simulink model "sm_robot_6legs_4bar"  (R2026a)
settings: Solver=ode15s  StopTime=33  MaxStep=1e-1  AbsTol=1e-4  EnableMultiTasking=on
PostLoadFcn:
  | sm_robot_6legs_4bar_param
undefined symbols (not defined in the file or in its folder): flr1_dep, flr1_len, flr1_wid, flr2_ang, flr2_dep, flr2_len, flr2_wid, flr3_dep, flr3_len, flr3_wid, flr_dep_pcnt, link_h, sigbuilder_block, X, Y, Z
libraries: Contact_Forces_Lib x24, sm_lib x12, nesl_utility x5, sm_robot_6legs_4bar_lib x2
CloseFcn:
  | try,close(h1_sm_robot_6legs_4bar),end
  | clear h1_sm_robot_6legs_4bar
  | 
  | clear simlog_sm_robot_6legs_4bar
  | clear logsout_sm_robot_6legs_4bar
Description:
  | Robot with Six Legs Built From 4 Four-Bar Linkages
  | 
  | Copyright 2026 The MathWorks, Inc.
settings Model: Creator=smiller  LastModifiedBy=smiller
settings DataIOCC: MaxDataPoints=20000  SignalLoggingName=logsout_sm_robot_6legs_4bar
settings DebuggingCC: PregeneratedLibrarySubsystemCodeDiagnostic=none
settings SimscapeCC: SimscapeNominalValues="[{\"value\":\"10\",\"unit\":\"V\"},{\"value\":\"1\",\"unit\":\"A\"},{\"value\":\"10\",\"unit\":\"N*m\"},{\"value\":\"10\",\"unit\":\"bar\"},{\"value\":\"100\",\"unit\":\"kJ/kg\"},{\"value\":\"1\",\"unit\":\"kW\"},{\"value\":\"300\",\"unit\":\"K\"},{\"value\":\"100\",\"unit\":\"cm^3/s\"},{\"value\":\"1\",\"unit\":\"kN\"},{\"value\":\"1\",\"unit\":\"g/cm^3\"},{\"value\":\"1\",\"unit\":\"l\"},{\"value\":\"1\",\"unit\":\"cm^2\"},{\"value\":\"60\",\"unit\":\"Hz\"}]"  SimscapeLogSimulationStatistics=on  SimscapeLogName=simlog_sm_robot_6legs_4bar  SimscapeLogDataHistory=20000.0
settings ConfigurationSet: Description=SimMechanics 2G
settings DiagnosticsConfigSet: SimMechanicsRigidlyBoundBlock=none
settings ExplorerConfigSet: InternalSimMechanicsExplorerSettings="<ExplorerConfiguration><canonicalview>default</canonicalview><AnimationSetting><BasePlaybackSpeed>1.0</BasePlaybackSpeed><PlaybackSpeedFactor>1.0</PlaybackSpeedFactor></AnimationSetting><TilePanel><TileInfo><Tiles Columns=\"2\" Count=\"3\" Rows=\"2\"><Column Weight=\"0.7315\"/><Column Weight=\"0.2685\"/><Row Weight=\"0.3085\"/><Row Weight=\"0.6915\"/><Tile Height=\"1\" Width=\"2\" X=\"0\" Y=\"0\"/><Tile Height=\"1\" Width=\"1\" X=\"0\" Y=\"1\"/><Tile Height=\"1\" Width=\"1\" X=\"1\" Y=\"1\"/></Tiles></TileInfo><SceneInfo><SceneViewer><BGColor><R>1</R><G>1</G><B>1</B></BGColor><Camera><DoPerspective>off</DoPerspective><Position><X>0.0595264996404310034</X><Y>0.0499787248889781988</Y><Z>-1.00000003287775163</Z></Position><Center><X>0.0595264996404310034</X><Y>0.0499787248889781988</Y><Z>-3.28777516322986685e-08</Z></Center><Up><X>0.00262045319823715674</X><Y>0.999996566606623727</Y><Z>0</Z></Up><ViewLimDist>1</ViewLimDist><YLim>0.107978090662275067</YLim><XLim>0.373654416059221617</XLim></Camera></SceneViewer><SceneViewer><BGColor><R>1</R><G>1</G><B>1</B></BGColor><Camera><DoPerspective>off</DoPerspective><Position><X>-0.747368609679726625</X><Y>0.501177725000622964</Y><Z>-0.454021615890128183</Z></Position><Center><X>0.0441835460138454428</X><Y>0.0596697074532213934</Y><Z>-0.0315102488735390512</Z></Center><Up><X>0.430303060009063654</X><Y>0.893614327868432756</Y><Z>0.127642898647299968</Z></Up><ViewLimDist>1</ViewLimDist><YLim>0.188959781718016667</YLim><XLim>0.209955313020018519</XLim></Camera></SceneViewer><SceneViewer><BGColor><R>1</R><G>1</G><B>1</B></BGColor><Camera><DoPerspective>off</DoPerspective><Position><X>0.0495837117205682534</X><Y>1.05623067821298733</Y><Z>0.0484295084377242974</Z></Position><Center><X>0.0433038677712018413</X><Y>0.0567676171677271926</Y><Z>0.0162712565261088245</Z></Center><Up><X>0.999975191574708711</X><Y>-0.00637917136590451708</Y><Z>0.00298703997456827193</Z></Up><ViewLimDist>1</ViewLimDist><YLim>0.384512045360850374</YLim><XLim>0.15427952437318071</XLim></Camera></SceneViewer></SceneInfo></TilePanel><MechEditorPanel><Cameras/><GfxPanelCameraMap/><VideoCreator><PlaybackSpeedRatio>2.0</PlaybackSpeedRatio><FrameRate>30</FrameRate><VideoFormat>MPEG-4</VideoFormat><FrameSize>auto</FrameSize></VideoCreator></MechEditorPanel></ExplorerConfiguration>"

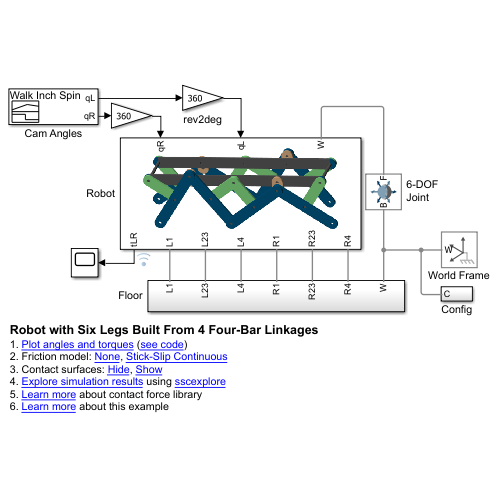
[thumbnail: Simulink's stored preview of the top-level diagram]
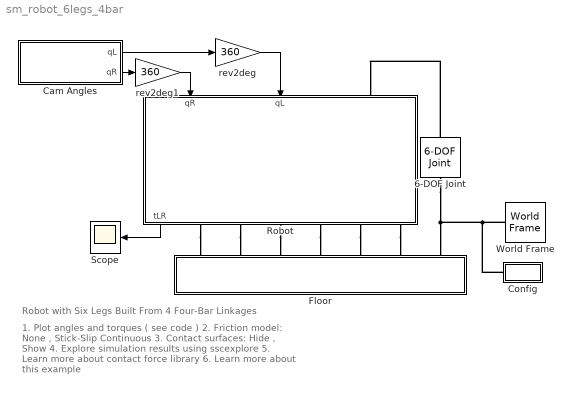
== system sm_robot_6legs_4bar ==
  note: Robot with Six Legs Built From 4 Four-Bar Linkages
  note: 1. Plot angles and torques ( see code )
      | 2. Friction model: None , Stick-Slip Continuous
      | 3. Contact surfaces: Hide , Show
      | 4. Explore simulation results using sscexplore
      | 5. Learn more about contact force library
      | 6. Learn more about this example
  6-DOF Joint : sm_lib/Joints/6-DOF Joint  JointMode=Normal  CompositeWrenchDir=FollowerOnBase  CompositeWrenchFrame=BaseFrame  SenseConstraintForce=off  SenseConstraintTorque=off  SenseTotalForce=off  SenseTotalTorque=off  PxPositionTargetSpecify=on  PxPositionTargetPriority=High  PxPositionTargetValue=-flr1_len/4-4.1e-2  PxPositionTargetValueUnits=m  PxVelocityTargetSpecify=off  PxVelocityTargetPriority=High  PxVelocityTargetValue=0  PxVelocityTargetValueUnits=m/s  PxEquilibriumPosition=0  PxEquilibriumPositionUnits=m  PxSpringStiffness=0  PxSpringStiffnessUnits=N/m  PxDampingCoefficient=0  PxDampingCoefficientUnits=N/(m/s)  PxLowerLimitSpecify=off  PxLowerLimitBound=-1  PxLowerLimitBoundUnits=m  PxLowerLimitStiffness=1e6  PxLowerLimitStiffnessUnits=N/m  PxLowerLimitDamping=1e3  PxLowerLimitDampingUnits=N/(m/s)  PxLowerLimitTransitionRegionWidth=1e-4  PxLowerLimitTransitionRegionWidthUnits=m  PxUpperLimitSpecify=off  PxUpperLimitBound=1  PxUpperLimitBoundUnits=m  PxUpperLimitStiffness=1e6  PxUpperLimitStiffnessUnits=N/m  PxUpperLimitDamping=1e3  PxUpperLimitDampingUnits=N/(m/s)  PxUpperLimitTransitionRegionWidth=1e-4  PxUpperLimitTransitionRegionWidthUnits=m  PxTorqueActuationMode=NoTorque  PxMotionActuationMode=ComputedMotion  PxSensePosition=off  PxSenseVelocity=off  PxSenseAcceleration=off  PxSenseTorqueForce=off  PxSenseLowerLimitTorqueForce=off  PxSenseUpperLimitTorqueForce=off  PyPositionTargetSpecify=on  PyPositionTargetPriority=High  PyPositionTargetValue=leg_l  PyPositionTargetValueUnits=m  PyVelocityTargetSpecify=off  PyVelocityTargetPriority=High  PyVelocityTargetValue=0  PyVelocityTargetValueUnits=m/s  PyEquilibriumPosition=0  PyEquilibriumPositionUnits=m  PySpringStiffness=0  PySpringStiffnessUnits=N/m  PyDampingCoefficient=0  PyDampingCoefficientUnits=N/(m/s)  PyLowerLimitSpecify=off  PyLowerLimitBound=-1  PyLowerLimitBoundUnits=m  PyLowerLimitStiffness=1e6  PyLowerLimitStiffnessUnits=N/m  PyLowerLimitDamping=1e3  PyLowerLimitDampingUnits=N/(m/s)  PyLowerLimitTransitionRegionWidth=1e-4  PyLowerLimitTransitionRegionWidthUnits=m  PyUpperLimitSpecify=off  PyUpperLimitBound=1  PyUpperLimitBoundUnits=m  PyUpperLimitStiffness=1e6  PyUpperLimitStiffnessUnits=N/m  PyUpperLimitDamping=1e3  PyUpperLimitDampingUnits=N/(m/s)  PyUpperLimitTransitionRegionWidth=1e-4  PyUpperLimitTransitionRegionWidthUnits=m  PyTorqueActuationMode=NoTorque  PyMotionActuationMode=ComputedMotion  PySensePosition=off  PySenseVelocity=off  PySenseAcceleration=off  PySenseTorqueForce=off  PySenseLowerLimitTorqueForce=off  PySenseUpperLimitTorqueForce=off  PzPositionTargetSpecify=off  PzPositionTargetPriority=High  PzPositionTargetValue=0  PzPositionTargetValueUnits=m  PzVelocityTargetSpecify=off  PzVelocityTargetPriority=High  PzVelocityTargetValue=0  PzVelocityTargetValueUnits=m/s  PzEquilibriumPosition=0  PzEquilibriumPositionUnits=m  PzSpringStiffness=0  PzSpringStiffnessUnits=N/m  PzDampingCoefficient=0  PzDampingCoefficientUnits=N/(m/s)  PzLowerLimitSpecify=off  PzLowerLimitBound=-1  PzLowerLimitBoundUnits=m  PzLowerLimitStiffness=1e6  PzLowerLimitStiffnessUnits=N/m  PzLowerLimitDamping=1e3  PzLowerLimitDampingUnits=N/(m/s)  PzLowerLimitTransitionRegionWidth=1e-4  PzLowerLimitTransitionRegionWidthUnits=m  PzUpperLimitSpecify=off  PzUpperLimitBound=1  PzUpperLimitBoundUnits=m  PzUpperLimitStiffness=1e6  PzUpperLimitStiffnessUnits=N/m  PzUpperLimitDamping=1e3  PzUpperLimitDampingUnits=N/(m/s)  PzUpperLimitTransitionRegionWidth=1e-4  PzUpperLimitTransitionRegionWidthUnits=m  PzTorqueActuationMode=NoTorque  PzMotionActuationMode=ComputedMotion  PzSensePosition=off  PzSenseVelocity=off  PzSenseAcceleration=off  PzSenseTorqueForce=off  PzSenseLowerLimitTorqueForce=off  PzSenseUpperLimitTorqueForce=off  SphPositionTargetSpecify=off  SphPositionTargetPriority=High  SphPositionTargetRotationMethod=None  SphPositionTargetFollAlignAxisA=+X  SphPositionTargetBaseAlignAxisA=+Y  SphPositionTargetFollAlignAxisB=+Y  SphPositionTargetBaseAlignAxisB=+Z  SphPositionTargetRotationStandardAxis=+Z  SphPositionTargetRotationAngle=0.0  SphPositionTargetRotationAngleUnits=deg  SphPositionTargetRotationArbitraryAxis=[0 0 1]  SphPositionTargetRotationSequenceAxes=FollowerAxes  SphPositionTargetRotationSequence=XYX  SphPositionTargetRotationSequenceAngles=[0 0 0]  SphPositionTargetRotationSequenceAnglesUnits=deg  SphPositionTargetRotationMatrix=[1 0 0; 0 1 0; 0 0 1]  SphPositionTargetQuaternion=[1 0 0 0]  SphVelocityTargetSpecify=off  SphVelocityTargetPriority=High  SphVelocityTargetValue=[0 0 0]  SphVelocityTargetValueUnits=deg/s  SphVelocityTargetInFollowerFrame=on  SphEqPosRotationMethod=None  SphEqPosFollAlignAxisA=+X  SphEqPosBaseAlignAxisA=+Y  SphEqPosFollAlignAxisB=+Y  SphEqPosBaseAlignAxisB=+Z  SphEqPosRotationStandardAxis=+Z  SphEqPosRotationAngle=0.0  SphEqPosRotationAngleUnits=deg  SphEqPosRotationArbitraryAxis=[0 0 1]  SphEqPosRotationSequenceAxes=FollowerAxes  SphEqPosRotationSequence=XYX  SphEqPosRotationSequenceAngles=[0 0 0]  SphEqPosRotationSequenceAnglesUnits=deg  SphEqPosRotationMatrix=[1 0 0; 0 1 0; 0 0 1]  SphEqPosQuaternion=[1 0 0 0]  SphSpringStiffness=0  SphSpringStiffnessUnits=N*m/deg  SphDampingCoefficient=0  SphDampingCoefficientUnits=N*m/(deg/s)  SphLowerLimitSpecify=off  SphLowerLimitBound=15  SphLowerLimitBoundUnits=deg  SphLowerLimitStiffness=1e4  SphLowerLimitStiffnessUnits=N*m/deg  SphLowerLimitDamping=10  SphLowerLimitDampingUnits=N*m/(deg/s)  SphLowerLimitTransitionRegionWidth=0.1  SphLowerLimitTransitionRegionWidthUnits=deg  SphUpperLimitSpecify=off  SphUpperLimitBound=45  SphUpperLimitBoundUnits=deg  SphUpperLimitStiffness=1e4  SphUpperLimitStiffnessUnits=N*m/deg  SphUpperLimitDamping=10  SphUpperLimitDampingUnits=N*m/(deg/s)  SphUpperLimitTransitionRegionWidth=0.1  SphUpperLimitTransitionRegionWidthUnits=deg  SphTorqueActuationMode=NoTorque  SphActuateTorqueX=off  SphActuateTorqueY=off  SphActuateTorqueZ=off  SphActuateTorque=off  SphActuationFrame=BaseFrame  SphSensePosition=off  SphSenseVelocityX=off  SphSenseVelocityY=off  SphSenseVelocityZ=off  SphSenseVelocity=off  SphSenseAccelerationX=off  SphSenseAccelerationY=off  SphSenseAccelerationZ=off  SphSenseAcceleration=off  SphSenseLowerLimitTorqueMag=off  SphSenseUpperLimitTorqueMag=off  SphSensingFrame=BaseFrame
  Cam Angles : Subsystem  Tag=STV Subsys  LoadFcn=sigbuilder_block('load');  StartFcn=sigbuilder_block('start');  StopFcn=sigbuilder_block('stop');  ClipboardFcn=sigbuilder_block('clipboard');  mask(Sigbuilder block){tuvar=[0:10]}
      mask help: Simulink:masks:SigbuilderBlock_MD
      mask init:
      | if ~strcmp(get_param(bdroot(gcbh),'SimulationStatus'),'stopped') tuvar = sigbuilder_block('maskInit'); end
      settings: CopyFcn=sigbuilder_block('copy');  DeleteFcn=sigbuilder_block('delete');  ModelCloseFcn=sigbuilder_block('modelClose');  PreSaveFcn=sigbuilder_block('preSave');  PauseFcn=sigbuilder_block('pause');  ContinueFcn=sigbuilder_block('continue');  NameChangeFcn=sigbuilder_block('namechange');  OpenFcn=sigbuilder_block('open',[355.8 216 550.8 400.2 ]);  CloseFcn=sigbuilder_block('close');
      mask Display: plot(0, 0, 100, 100,[2, 2, 32, 32, 2], [68, 8, 8, 68, 68],[32, 2], [38, 38], [32, 19, 2],[53, 60, 44], [32, 17, 17, 2],[16, 16, 31, 31]);txt = getActiveGroup(gcbh);text(2, 100, txt,'verticalAlignment', 'top');
  Config : Subsystem
  Floor : Subsystem
  Robot : Subsystem  Tag=PublishSubsystem
      mask Display: image('sm_robot_6legs_4bar_robot_IMAGE.png')
  Scope : Scope
      settings: ActiveDisplayYMinimum=-0.58589  ActiveDisplayYMaximum=0.586
  World Frame : sm_lib/Frames and Transforms/World Frame
  rev2deg : Gain  Gain=360
  rev2deg1 : Gain  Gain=360
  wires:
  Cam Angles/2(qR) -> rev2deg1/1
  Cam Angles/1(qL) -> rev2deg/1
  Robot/1(tLR) -> Scope/1
  rev2deg/1 -> Robot/2(qL)
  rev2deg1/1 -> Robot/1(qR)
  connections:
  World Frame/RConn1 -- Config/LConn1 -- 6-DOF Joint/LConn1 -- Floor/LConn7
  6-DOF Joint/RConn1 -- Robot/LConn1
  Robot/RConn4 -- Floor/LConn4
  Robot/RConn5 -- Floor/LConn5
  Robot/RConn6 -- Floor/LConn6
  Robot/RConn1 -- Floor/LConn1
  Robot/RConn2 -- Floor/LConn2
  Robot/RConn3 -- Floor/LConn3

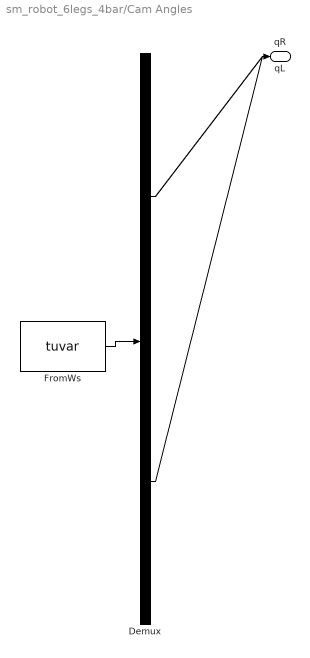
== system sm_robot_6legs_4bar/Cam Angles ==
  Demux : Demux  Tag=STV Demux  Outputs=2
      settings: DisplayOption=none
  FromWs : FromWorkspace  Tag=STV FromWs  VariableName=tuvar
      SigBuilderData=|
      | common.afterFinalStr = 'Extrapolate'
      | common.sampleTime = 0
      | dataSet(1).timeRange = [0 35]
      | dataSet(1).name = 'Walk Inch Spin'
      | dataSet(2).timeRange = [0 30]
      | dataSet(2).name = 'Walk'
      | dataSet(3).timeRange = [0 30]
      | dataSet(3).name = 'Inchworm'
      | sbobj.Groups(1).Name = 'Walk Inch Spin'
      | sbobj.Groups(1).Signals(1).Name = 'qL'
      | sbobj.Groups(1).Signals(1).XData = [0 0.5 3 3.5 5 5.5 25.5 26 28 28.5 32.5 35]
      | sbobj.Groups(1).Signals(1).YData = [0.75 0.75 1.75 1.75 2.25 2.25 12.25 12.25 12.75 12.75 14.75 14.75]
      | sbobj.Groups(1).Signals(2).Name = 'qR'
      | sbobj.Groups(1).Signals(2).XData = [0 0.5 3 5 5.5 25.5 28.5 32.5 35]
      | sbobj.Groups(1).Signals(2).YData = [0.25 0.25 1.25 1.25 1.25 11.25 11.25 9.25 9.25]
      | sbobj.Groups(1).TimeRange = [0 35]
      | sbobj.Groups(2).Name = 'Walk'
      | sbobj.Groups(2).Signals(1).Name = 'qL'
      | sbobj.Groups(2).Signals(1).XData = [0 1 22 30]
      | sbobj.Groups(2).Signals(1).YData = [0.75 0.75 11.75 11.75]
      | sbobj.Groups(2).Signals(2).Name = 'qR'
      | sbobj.Groups(2).Signals(2).XData = [0 1 22 30]
      | sbobj.Groups(2).Signals(2).YData = [0.25 0.25 11.25 11.25]
      | sbobj.Groups(2).TimeRange = [0 30]
      | sbobj.Groups(3).Name = 'Inchworm'
      | sbobj.Groups(3).Signals(1).Name = 'qL'
      | sbobj.Groups(3).Signals(1).XData = [0 1 22 30]
      | sbobj.Groups(3).Signals(1).YData = [0.75 0.75 11.75 11.75]
      | sbobj.Groups(3).Signals(2).Name = 'qR'
      | sbobj.Groups(3).Signals(2).XData = [0 1 22 30]
      | sbobj.Groups(3).Signals(2).YData = [0.75 0.75 11.75 11.75]
      | sbobj.Groups(3).TimeRange = [0 30]
  qL : Outport  Tag=STV Outport  VectorParamsAs1DForOutWhenUnconnected=off
  qR : Outport  Tag=STV Outport  Port=2  VectorParamsAs1DForOutWhenUnconnected=off
  wires:
  FromWs/1 -> Demux/1
  Demux/1 -> qL/1
  Demux/2 -> qR/1

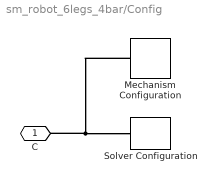
== system sm_robot_6legs_4bar/Config ==
  Mechanism Configuration : sm_lib/Utilities/Mechanism Configuration  UniformGravity=Constant  GravityVector=[0 -9.80665 0]  GravityVectorUnits=m/s^2  LinearizationDelta=0.001  JointModeTransitionNonlinearIterations=2
  Solver Configuration : nesl_utility/Solver Configuration  PhysicalDomain=network_engine_domain  SubClassName=solver  LeftPortType=input  RightPortType=generic  Tones=[]  Harmonics=[]  SimulateNoise=off  Profile=off  UseLocalSampling=off  EnableSwitchedLinearOptims=on  FrequencyDomain=off  UseCCode=off  RelTol=0.001  AbsTol=1e-06  MinStep=1e-09  ToWorkspace=off  RevertToSquareIcSolve=off  NumHomotopyIterations=100  PhasorMode=off  PhasorModeNumHarmonics=1  ConsistencySolver=NEWTON_FTOL  CanonicalOrdering=UNORDERED  OptimizeIntermediates=UNOPTIMIZED  IndexReductionMethod=DerivativeReplacement  DoDC=off  ResidualTolerance=1e-09  ConsistencyTolSource=GLOBAL  ConsistencyAbsTol=0.001  ConsistencyRelTol=0.001  ConsistencyTolFactor=0.001  UseLocalSolver=off  LocalSolverChoice=NE_BACKWARD_EULER_ADVANCER  ResolveIndetEquations=on  FunctionEvalNumThread=1  LocalSolverSampleTime=0.001  DoFixedCost=off  MaxNonlinIter=3  MaxModeIter=2  ComputeImpulses=off  ImpulseIterations=2  LinearAlgebra=Sparse  LinearAlgebraNumThread=0  EquationFormulation=NE_TIME_EF  DelaysMemoryBudget=1024  AutomaticFiltering=on  FilteringTimeConstant=0.001  PartitionStorageMethod=AS_NEEDED  PartitionMemoryBudget=1024  PartitionMethod=FAST  MultibodyUseLocalSolver=off  MultibodyLocalSolverChoice=ODE1  MultibodyLocalSolverSampleTime=0.001
  C : PMIOPort  Side=Left
  connections:
  Mechanism Configuration/RConn1 -- C/RConn1 -- Solver Configuration/RConn1

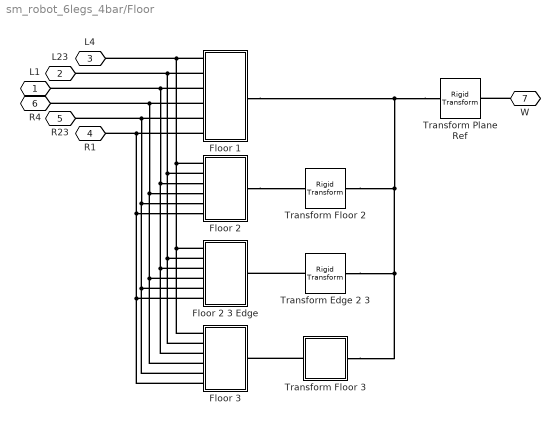
== system sm_robot_6legs_4bar/Floor ==
  Floor 1 : Subsystem  Tag=PublishSubsystem
  Floor 2 : Subsystem
  Floor 2 3 Edge : Subsystem
  Floor 3 : Subsystem
  Transform Edge 2 3 : sm_lib/Frames and Transforms/Rigid Transform  RotationMethod=AlignedAxes  FollAlignAxisA=+Z  BaseAlignAxisA=+Y  FollAlignAxisB=+X  BaseAlignAxisB=+Z  RotationStandardAxis=+Y  RotationAngle=-10  RotationAngleUnits=deg  RotationArbitraryAxis=[0 0 1]  RotationSequenceAxes=FollowerAxes  RotationSequence=XYX  RotationSequenceAngles=[0 0 0]  RotationSequenceAnglesUnits=deg  RotationMatrix=[1 0 0; 0 1 0; 0 0 1]  Quaternion=[1 0 0 0]  TranslationMethod=Cartesian  TranslationCartesianOffset=[cosd(flr2_ang) 0 sind(flr2_ang)]*flr2_len  TranslationCartesianOffsetUnits=m  TranslationStandardAxis=+Z  TranslationStandardOffset=0  TranslationStandardOffsetUnits=m  TranslationROffset=0  TranslationROffsetUnits=m  TranslationThetaOffset=0  TranslationThetaOffsetUnits=deg  TranslationZOffset=0  TranslationZOffsetUnits=m
  Transform Floor 2 : sm_lib/Frames and Transforms/Rigid Transform  RotationMethod=StandardAxis  FollAlignAxisA=+X  BaseAlignAxisA=+Y  FollAlignAxisB=+Y  BaseAlignAxisB=+Z  RotationStandardAxis=+Y  RotationAngle=-flr2_ang  RotationAngleUnits=deg  RotationArbitraryAxis=[0 0 1]  RotationSequenceAxes=FollowerAxes  RotationSequence=XYX  RotationSequenceAngles=[0 0 0]  RotationSequenceAnglesUnits=deg  RotationMatrix=[1 0 0; 0 1 0; 0 0 1]  Quaternion=[1 0 0 0]  TranslationMethod=Cartesian  TranslationCartesianOffset=[cosd(flr2_ang) 0 sind(flr2_ang)]*flr2_len/2  TranslationCartesianOffsetUnits=m  TranslationStandardAxis=+Z  TranslationStandardOffset=0  TranslationStandardOffsetUnits=m  TranslationROffset=0  TranslationROffsetUnits=m  TranslationThetaOffset=0  TranslationThetaOffsetUnits=deg  TranslationZOffset=0  TranslationZOffsetUnits=m
  Transform Floor 3 : Subsystem
  Transform Plane Ref : sm_lib/Frames and Transforms/Rigid Transform  RotationMethod=StandardAxis  FollAlignAxisA=+X  BaseAlignAxisA=+Y  FollAlignAxisB=+Y  BaseAlignAxisB=+Z  RotationStandardAxis=+X  RotationAngle=-90  RotationAngleUnits=deg  RotationArbitraryAxis=[0 0 1]  RotationSequenceAxes=FollowerAxes  RotationSequence=XYX  RotationSequenceAngles=[0 0 0]  RotationSequenceAnglesUnits=deg  RotationMatrix=[1 0 0; 0 1 0; 0 0 1]  Quaternion=[1 0 0 0]  TranslationMethod=None  TranslationCartesianOffset=[0 0 0]  TranslationCartesianOffsetUnits=m  TranslationStandardAxis=+Z  TranslationStandardOffset=0  TranslationStandardOffsetUnits=m  TranslationROffset=0  TranslationROffsetUnits=m  TranslationThetaOffset=0  TranslationThetaOffsetUnits=deg  TranslationZOffset=0  TranslationZOffsetUnits=m
  L1 : PMIOPort  Side=Left
  L23 : PMIOPort  Port=2  Side=Left
  L4 : PMIOPort  Port=3  Side=Left
  R1 : PMIOPort  Port=4  Side=Left
  R23 : PMIOPort  Port=5  Side=Left
  R4 : PMIOPort  Port=6  Side=Left
  W : PMIOPort  Port=7  Side=Left
  connections:
  W/RConn1 -- Transform Plane Ref/LConn1
  Floor 3/LConn1 -- Floor 2 3 Edge/LConn1 -- Floor 1/LConn1 -- L4/RConn1 -- Floor 2/LConn1
  Floor 3/LConn2 -- Floor 2 3 Edge/LConn2 -- Floor 1/LConn2 -- L23/RConn1 -- Floor 2/LConn2
  Floor 3/LConn3 -- Floor 2/LConn3 -- Floor 1/LConn3 -- L1/RConn1 -- Floor 2 3 Edge/LConn3
  R4/RConn1 -- Floor 1/LConn4 -- Floor 2 3 Edge/LConn4 -- Floor 3/LConn4 -- Floor 2/LConn4
  Transform Plane Ref/RConn1 -- Floor 1/RConn1 -- Transform Floor 3/LConn1 -- Transform Edge 2 3/LConn1 -- Transform Floor 2/LConn1
  R23/RConn1 -- Floor 1/LConn5 -- Floor 2 3 Edge/LConn5 -- Floor 3/LConn5 -- Floor 2/LConn5
  Floor 3/LConn6 -- Floor 2 3 Edge/LConn6 -- Floor 1/LConn6 -- R1/RConn1 -- Floor 2/LConn6
  Floor 2/RConn1 -- Transform Floor 2/RConn1
  Transform Floor 3/RConn1 -- Floor 3/RConn1
  Transform Edge 2 3/RConn1 -- Floor 2 3 Edge/RConn1

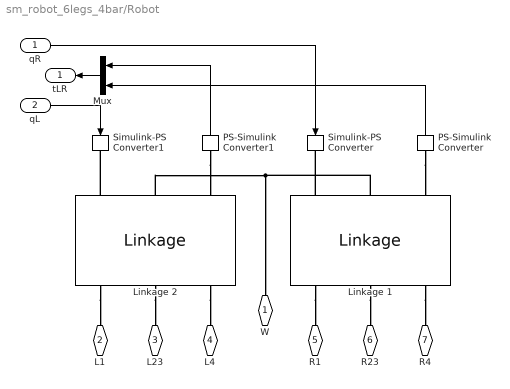
== system sm_robot_6legs_4bar/Robot ==
  qR : Inport
  qL : Inport  Port=2
  Linkage 1 : sm_robot_6legs_4bar_lib/Linkage  popup_LorR=Right
      link override Cam L12/Rod: popup_zori=Local +Z
      link override Cam L34/Rod: popup_zori=Local +Z
      link override Frame/Rod F1: popup_zori=Local +Z
      link override Frame/Rod F5: popup_zori=Local +Z
      link override Frame/Rod H1: popup_zori=Local +Z
      link override Frame/Rod H2: popup_zori=Local +Z
      link override Frame/Rod H4: popup_zori=Local +Z
      link override Frame/Rod H5: popup_zori=Local +Z
      link override Frame/Rod5 H3: popup_zori=Local +Z
      link override Leg L1/Rod: popup_zori=Local +Z
      link override Leg L3/Rod B: popup_zori=Local +Z
      link override Leg L3/Rod C: popup_zori=Local +Z
      link override Leg L3/Rod F: popup_zori=Local +Z
      link override Link L1/Rod: popup_zori=Local +Z
      link override Link L2/Rod: popup_zori=Local +Z
      link override Link L3/Rod: popup_zori=Local +Z
      link override Link L4/Rod: popup_zori=Local +Z
      settings: AttributesFormatString=%<popup_LorR>
  Linkage 2 : sm_robot_6legs_4bar_lib/Linkage  Tag=PublishSubsystem  popup_LorR=Left
      link override Cam L12/Rod: popup_zori=Local -Z
      link override Cam L34/Rod: popup_zori=Local -Z
      link override Frame/Rod F1: popup_zori=Local -Z
      link override Frame/Rod F5: popup_zori=Local -Z
      link override Frame/Rod H1: popup_zori=Local -Z
      link override Frame/Rod H2: popup_zori=Local -Z
      link override Frame/Rod H4: popup_zori=Local -Z
      link override Frame/Rod H5: popup_zori=Local -Z
      link override Frame/Rod5 H3: popup_zori=Local -Z
      link override Leg L1/Rod: popup_zori=Local -Z
      link override Leg L3/Rod B: popup_zori=Local -Z
      link override Leg L3/Rod C: popup_zori=Local -Z
      link override Leg L3/Rod F: popup_zori=Local -Z
      link override Link L1/Rod: popup_zori=Local -Z
      link override Link L2/Rod: popup_zori=Local -Z
      link override Link L3/Rod: popup_zori=Local -Z
      link override Link L4/Rod: popup_zori=Local -Z
      settings: AttributesFormatString=%<popup_LorR>
  Mux : Mux  Inputs=2
  PS-Simulink Converter : nesl_utility/PS-Simulink Converter  PhysicalDomain=network_engine_domain  SubClassName=ps_output  LeftPortType=input  RightPortType=output  PseudoPeriodic=off  Frequencies=[]  VectorFormat=1-D array  Unit=1  AffineConversion=off
  PS-Simulink Converter1 : nesl_utility/PS-Simulink Converter  PhysicalDomain=network_engine_domain  SubClassName=ps_output  LeftPortType=input  RightPortType=output  PseudoPeriodic=off  Frequencies=[]  VectorFormat=1-D array  Unit=1  AffineConversion=off
  Simulink-PS Converter : nesl_utility/Simulink-PS Converter  PhysicalDomain=network_engine_domain  SubClassName=ps_input  LeftPortType=input  RightPortType=output  PseudoPeriodic=off  Frequencies=[]  NoiseDistribution=none  NoiseParameters=[]  Unit=deg  AffineConversion=off  FilteringAndDerivatives=filter  SimscapeFilterOrder=2  InputFilterTimeConstant=0.005  UdotUserProvided=0
  Simulink-PS Converter1 : nesl_utility/Simulink-PS Converter  PhysicalDomain=network_engine_domain  SubClassName=ps_input  LeftPortType=input  RightPortType=output  PseudoPeriodic=off  Frequencies=[]  NoiseDistribution=none  NoiseParameters=[]  Unit=deg  AffineConversion=off  FilteringAndDerivatives=filter  SimscapeFilterOrder=2  InputFilterTimeConstant=0.005  UdotUserProvided=0
  W : PMIOPort  Side=Left
  L1 : PMIOPort  Port=2  Side=Right
  L23 : PMIOPort  Port=3  Side=Right
  L4 : PMIOPort  Port=4  Side=Right
  R1 : PMIOPort  Port=5  Side=Right
  R23 : PMIOPort  Port=6  Side=Right
  R4 : PMIOPort  Port=7  Side=Right
  tLR : Outport  VectorParamsAs1DForOutWhenUnconnected=off
  wires:
  PS-Simulink Converter/1 -> Mux/2
  PS-Simulink Converter1/1 -> Mux/1
  Mux/1 -> tLR/1
  qL/1 -> Simulink-PS Converter1/1
  qR/1 -> Simulink-PS Converter/1
  connections:
  Linkage 2/LConn1 -- Simulink-PS Converter1/RConn1
  Linkage 2/RConn1 -- L1/RConn1
  PS-Simulink Converter1/LConn1 -- Linkage 2/LConn3
  PS-Simulink Converter/LConn1 -- Linkage 1/LConn3
  Linkage 1/LConn1 -- Simulink-PS Converter/RConn1
  Linkage 2/LConn2 -- Linkage 1/LConn2 -- W/RConn1
  Linkage 2/RConn3 -- L4/RConn1
  Linkage 2/RConn2 -- L23/RConn1
  Linkage 1/RConn3 -- R4/RConn1
  Linkage 1/RConn1 -- R1/RConn1
  Linkage 1/RConn2 -- R23/RConn1

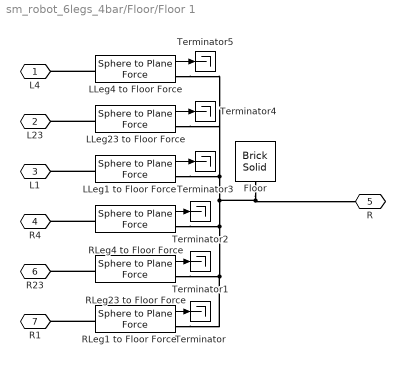
== system sm_robot_6legs_4bar/Floor/Floor 1 ==
  Floor : sm_lib/Body Elements/Brick Solid  BrickDimensions=[flr1_len flr1_wid flr1_dep]  BrickDimensionsUnits=m  ExportEntireGeometry=off  InertiaType=CalculateFromGeometry  BasedOnType=Density  Density=1000  DensityUnits=kg/m^3  Mass=1  MassUnits=kg  CenterOfMass=[0 0 0]  CenterOfMassUnits=m  MomentsOfInertia=[1 1 1]  MomentsOfInertiaUnits=kg*m^2  ProductsOfInertia=[0 0 0]  ProductsOfInertiaUnits=kg*m^2  GraphicType=FromGeometry  MarkerShape=Sphere  MarkerSize=10  GraphicVisPropType=SimpleVisualProperties  GraphicDiffuseColor=flr_clr  GraphicOpacity=1.0  GraphicSpecularColor=[0.5 0.5 0.5 1.0]  GraphicAmbientColor=[0.15 0.15 0.15 1.0]  GraphicEmissiveColor=[0.0 0.0 0.0 1.0]  GraphicShininess=75  DoExposeReferenceFrame=on  SerializedFrames=<Frames/>
  LLeg1 to Floor Force : Contact_Forces_Lib/3D/Sphere to Plane Force  sphere_rad=link_h/2  plane_lenx=flr1_len  plane_leny=flr1_wid  plane_depth=flr1_dep/2  force_law=Linear  k_contact=flr_k  b_contact=flr_b  pen_full_damp_F=1e-4  pen_exponent=1  custom_param_1=1  custom_param_2=1  friction_law=Stick-Slip Continuous  mu_kinetic=flr_muk  mu_static=flr_mus  v_thr=flr_vth  vis_on=off  vis_opc_en=0  vis_len_plaBz=flr1_dep*flr_dep_pcnt  vis_clr=[0.9 0.2 0.2]  vis_opc=0.7
  LLeg23 to Floor Force : Contact_Forces_Lib/3D/Sphere to Plane Force  sphere_rad=link_h/2  plane_lenx=flr1_len  plane_leny=flr1_wid  plane_depth=flr1_dep/2  force_law=Linear  k_contact=flr_k  b_contact=flr_b  pen_full_damp_F=1e-4  pen_exponent=1  custom_param_1=1  custom_param_2=1  friction_law=Stick-Slip Continuous  mu_kinetic=flr_muk  mu_static=flr_mus  v_thr=flr_vth  vis_on=off  vis_opc_en=0  vis_len_plaBz=flr1_dep*flr_dep_pcnt  vis_clr=[0.9 0.2 0.2]  vis_opc=0.7
  LLeg4 to Floor Force : Contact_Forces_Lib/3D/Sphere to Plane Force  sphere_rad=link_h/2  plane_lenx=flr1_len  plane_leny=flr1_wid  plane_depth=flr1_dep/2  force_law=Linear  k_contact=flr_k  b_contact=flr_b  pen_full_damp_F=1e-4  pen_exponent=1  custom_param_1=1  custom_param_2=1  friction_law=Stick-Slip Continuous  mu_kinetic=flr_muk  mu_static=flr_mus  v_thr=flr_vth  vis_on=off  vis_opc_en=0  vis_len_plaBz=flr1_dep*flr_dep_pcnt  vis_clr=[0.9 0.2 0.2]  vis_opc=0.7
  RLeg1 to Floor Force : Contact_Forces_Lib/3D/Sphere to Plane Force  sphere_rad=link_h/2  plane_lenx=flr1_len  plane_leny=flr1_wid  plane_depth=flr1_dep/2  force_law=Linear  k_contact=flr_k  b_contact=flr_b  pen_full_damp_F=1e-4  pen_exponent=1  custom_param_1=1  custom_param_2=1  friction_law=Stick-Slip Continuous  mu_kinetic=flr_muk  mu_static=flr_mus  v_thr=flr_vth  vis_on=off  vis_opc_en=0  vis_len_plaBz=flr1_dep*flr_dep_pcnt  vis_clr=[0.9 0.2 0.2]  vis_opc=0.7
  RLeg23 to Floor Force : Contact_Forces_Lib/3D/Sphere to Plane Force  sphere_rad=link_h/2  plane_lenx=flr1_len  plane_leny=flr1_wid  plane_depth=flr1_dep/2  force_law=Linear  k_contact=flr_k  b_contact=flr_b  pen_full_damp_F=1e-4  pen_exponent=1  custom_param_1=1  custom_param_2=1  friction_law=Stick-Slip Continuous  mu_kinetic=flr_muk  mu_static=flr_mus  v_thr=flr_vth  vis_on=off  vis_opc_en=0  vis_len_plaBz=flr1_dep*flr_dep_pcnt  vis_clr=[0.9 0.2 0.2]  vis_opc=0.7
  RLeg4 to Floor Force : Contact_Forces_Lib/3D/Sphere to Plane Force  sphere_rad=link_h/2  plane_lenx=flr1_len  plane_leny=flr1_wid  plane_depth=flr1_dep/2  force_law=Linear  k_contact=flr_k  b_contact=flr_b  pen_full_damp_F=1e-4  pen_exponent=1  custom_param_1=1  custom_param_2=1  friction_law=Stick-Slip Continuous  mu_kinetic=flr_muk  mu_static=flr_mus  v_thr=flr_vth  vis_on=off  vis_opc_en=0  vis_len_plaBz=flr1_dep*flr_dep_pcnt  vis_clr=[0.9 0.2 0.2]  vis_opc=0.7
  Terminator{,1..5} (6 alike) : Terminator
  L4 : PMIOPort  Side=Left
  L23 : PMIOPort  Port=2  Side=Left
  L1 : PMIOPort  Port=3  Side=Left
  R4 : PMIOPort  Port=4  Side=Left
  R : PMIOPort  Port=5  Side=Right
  R23 : PMIOPort  Port=6  Side=Left
  R1 : PMIOPort  Port=7  Side=Left
  wires:
  RLeg1 to Floor Force/1 -> Terminator/1
  LLeg23 to Floor Force/1 -> Terminator4/1
  LLeg4 to Floor Force/1 -> Terminator5/1
  LLeg1 to Floor Force/1 -> Terminator3/1
  RLeg4 to Floor Force/1 -> Terminator2/1
  RLeg23 to Floor Force/1 -> Terminator1/1
  connections:
  Floor/RConn1 -- R/RConn1 -- RLeg23 to Floor Force/RConn1 -- RLeg1 to Floor Force/RConn1 -- RLeg4 to Floor Force/RConn1 -- LLeg1 to Floor Force/RConn1 -- LLeg23 to Floor Force/RConn1 -- LLeg4 to Floor Force/RConn1
  LLeg23 to Floor Force/LConn1 -- L23/RConn1
  RLeg1 to Floor Force/LConn1 -- R1/RConn1
  RLeg23 to Floor Force/LConn1 -- R23/RConn1
  RLeg4 to Floor Force/LConn1 -- R4/RConn1
  LLeg1 to Floor Force/LConn1 -- L1/RConn1
  LLeg4 to Floor Force/LConn1 -- L4/RConn1

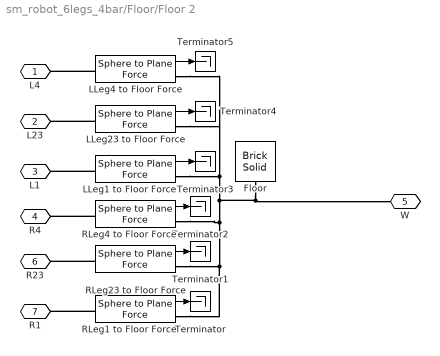
== system sm_robot_6legs_4bar/Floor/Floor 2 ==
  Floor : sm_lib/Body Elements/Brick Solid  BrickDimensions=[flr2_len flr2_wid flr2_dep]  BrickDimensionsUnits=m  ExportEntireGeometry=off  InertiaType=CalculateFromGeometry  BasedOnType=Density  Density=1000  DensityUnits=kg/m^3  Mass=1  MassUnits=kg  CenterOfMass=[0 0 0]  CenterOfMassUnits=m  MomentsOfInertia=[1 1 1]  MomentsOfInertiaUnits=kg*m^2  ProductsOfInertia=[0 0 0]  ProductsOfInertiaUnits=kg*m^2  GraphicType=FromGeometry  MarkerShape=Sphere  MarkerSize=10  GraphicVisPropType=SimpleVisualProperties  GraphicDiffuseColor=flr_clr  GraphicOpacity=1.0  GraphicSpecularColor=[0.5 0.5 0.5 1.0]  GraphicAmbientColor=[0.15 0.15 0.15 1.0]  GraphicEmissiveColor=[0.0 0.0 0.0 1.0]  GraphicShininess=75  DoExposeReferenceFrame=on  SerializedFrames=<Frames/>
  LLeg1 to Floor Force : Contact_Forces_Lib/3D/Sphere to Plane Force  sphere_rad=link_h/2  plane_lenx=flr2_len  plane_leny=flr2_wid  plane_depth=flr2_dep/2  force_law=Linear  k_contact=flr_k  b_contact=flr_b  pen_full_damp_F=1e-4  pen_exponent=1  custom_param_1=1  custom_param_2=1  friction_law=Stick-Slip Continuous  mu_kinetic=flr_muk  mu_static=flr_mus  v_thr=flr_vth  vis_on=off  vis_opc_en=0  vis_len_plaBz=flr2_dep*flr_dep_pcnt  vis_clr=[0.9 0.2 0.2]  vis_opc=0.7
  LLeg23 to Floor Force : Contact_Forces_Lib/3D/Sphere to Plane Force  sphere_rad=link_h/2  plane_lenx=flr2_len  plane_leny=flr2_wid  plane_depth=flr2_dep/2  force_law=Linear  k_contact=flr_k  b_contact=flr_b  pen_full_damp_F=1e-4  pen_exponent=1  custom_param_1=1  custom_param_2=1  friction_law=Stick-Slip Continuous  mu_kinetic=flr_muk  mu_static=flr_mus  v_thr=flr_vth  vis_on=off  vis_opc_en=0  vis_len_plaBz=flr2_dep*flr_dep_pcnt  vis_clr=[0.9 0.2 0.2]  vis_opc=0.7
  LLeg4 to Floor Force : Contact_Forces_Lib/3D/Sphere to Plane Force  sphere_rad=link_h/2  plane_lenx=flr2_len  plane_leny=flr2_wid  plane_depth=flr2_dep/2  force_law=Linear  k_contact=flr_k  b_contact=flr_b  pen_full_damp_F=1e-4  pen_exponent=1  custom_param_1=1  custom_param_2=1  friction_law=Stick-Slip Continuous  mu_kinetic=flr_muk  mu_static=flr_mus  v_thr=flr_vth  vis_on=off  vis_opc_en=0  vis_len_plaBz=flr2_dep*flr_dep_pcnt  vis_clr=[0.9 0.2 0.2]  vis_opc=0.7
  RLeg1 to Floor Force : Contact_Forces_Lib/3D/Sphere to Plane Force  sphere_rad=link_h/2  plane_lenx=flr2_len  plane_leny=flr2_wid  plane_depth=flr2_dep/2  force_law=Linear  k_contact=flr_k  b_contact=flr_b  pen_full_damp_F=1e-4  pen_exponent=1  custom_param_1=1  custom_param_2=1  friction_law=Stick-Slip Continuous  mu_kinetic=flr_muk  mu_static=flr_mus  v_thr=flr_vth  vis_on=off  vis_opc_en=0  vis_len_plaBz=flr2_dep*flr_dep_pcnt  vis_clr=[0.9 0.2 0.2]  vis_opc=0.7
  RLeg23 to Floor Force : Contact_Forces_Lib/3D/Sphere to Plane Force  sphere_rad=link_h/2  plane_lenx=flr2_len  plane_leny=flr2_wid  plane_depth=flr2_dep/2  force_law=Linear  k_contact=flr_k  b_contact=flr_b  pen_full_damp_F=1e-4  pen_exponent=1  custom_param_1=1  custom_param_2=1  friction_law=Stick-Slip Continuous  mu_kinetic=flr_muk  mu_static=flr_mus  v_thr=flr_vth  vis_on=off  vis_opc_en=0  vis_len_plaBz=flr2_dep*flr_dep_pcnt  vis_clr=[0.9 0.2 0.2]  vis_opc=0.7
  RLeg4 to Floor Force : Contact_Forces_Lib/3D/Sphere to Plane Force  sphere_rad=link_h/2  plane_lenx=flr2_len  plane_leny=flr2_wid  plane_depth=flr2_dep/2  force_law=Linear  k_contact=flr_k  b_contact=flr_b  pen_full_damp_F=1e-4  pen_exponent=1  custom_param_1=1  custom_param_2=1  friction_law=Stick-Slip Continuous  mu_kinetic=flr_muk  mu_static=flr_mus  v_thr=flr_vth  vis_on=off  vis_opc_en=0  vis_len_plaBz=flr2_dep*flr_dep_pcnt  vis_clr=[0.9 0.2 0.2]  vis_opc=0.7
  Terminator{,1..5} (6 alike) : Terminator
  L4 : PMIOPort  Side=Left
  L23 : PMIOPort  Port=2  Side=Left
  L1 : PMIOPort  Port=3  Side=Left
  R4 : PMIOPort  Port=4  Side=Left
  W : PMIOPort  Port=5  Side=Right
  R23 : PMIOPort  Port=6  Side=Left
  R1 : PMIOPort  Port=7  Side=Left
  wires:
  RLeg23 to Floor Force/1 -> Terminator1/1
  RLeg4 to Floor Force/1 -> Terminator2/1
  LLeg1 to Floor Force/1 -> Terminator3/1
  LLeg4 to Floor Force/1 -> Terminator5/1
  LLeg23 to Floor Force/1 -> Terminator4/1
  RLeg1 to Floor Force/1 -> Terminator/1
  connections:
  LLeg4 to Floor Force/LConn1 -- L4/RConn1
  LLeg1 to Floor Force/LConn1 -- L1/RConn1
  RLeg4 to Floor Force/LConn1 -- R4/RConn1
  RLeg23 to Floor Force/LConn1 -- R23/RConn1
  RLeg1 to Floor Force/LConn1 -- R1/RConn1
  LLeg23 to Floor Force/LConn1 -- L23/RConn1
  Floor/RConn1 -- W/RConn1 -- LLeg4 to Floor Force/RConn1 -- LLeg23 to Floor Force/RConn1 -- LLeg1 to Floor Force/RConn1 -- RLeg4 to Floor Force/RConn1 -- RLeg1 to Floor Force/RConn1 -- RLeg23 to Floor Force/RConn1

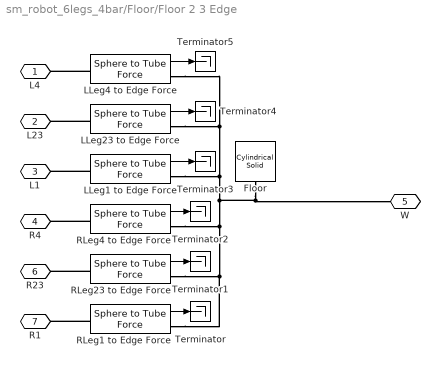
== system sm_robot_6legs_4bar/Floor/Floor 2 3 Edge ==
  Floor : sm_lib/Body Elements/Cylindrical Solid  CylinderRadius=flr2_dep/2  CylinderRadiusUnits=m  CylinderLength=flr2_wid  CylinderLengthUnits=m  ExportEntireGeometry=off  InertiaType=CalculateFromGeometry  BasedOnType=Density  Density=1000  DensityUnits=kg/m^3  Mass=1  MassUnits=kg  CenterOfMass=[0 0 0]  CenterOfMassUnits=m  MomentsOfInertia=[1 1 1]  MomentsOfInertiaUnits=kg*m^2  ProductsOfInertia=[0 0 0]  ProductsOfInertiaUnits=kg*m^2  GraphicType=FromGeometry  MarkerShape=Sphere  MarkerSize=10  GraphicVisPropType=SimpleVisualProperties  GraphicDiffuseColor=flr_clr  GraphicOpacity=1.0  GraphicSpecularColor=[0.5 0.5 0.5 1.0]  GraphicAmbientColor=[0.15 0.15 0.15 1.0]  GraphicEmissiveColor=[0.0 0.0 0.0 1.0]  GraphicShininess=75  DoExposeReferenceFrame=on  SerializedFrames=<Frames/>
  LLeg1 to Edge Force : Contact_Forces_Lib/3D/Sphere to Tube Force  radius_sphere=link_h/2  radius_tube=flr2_dep/2*(1-0.1)  d_tube=flr2_dep/2*(2*0.1)  l_tube=flr2_wid  active_angle=[-flr2_ang 0]  force_law=Linear  k_contact=flr_k  b_contact=flr_b  pen_full_damp_F=1e-4  pen_exponent=1  custom_param_1=1  custom_param_2=1  friction_law=Stick-Slip Continuous  mu_kinetic=flr_muk  mu_static=flr_mus  v_thr=flr_vth  vis_on=off  vis_opc_en=0  vis_len_tubBx=flr2_dep*flr_dep_pcnt  vis_clr=[0.9 0.2 0.2]  vis_opc=0.7
      settings: SourceProductName=Simscape Multibody Contact Forces Library
  LLeg23 to Edge Force : Contact_Forces_Lib/3D/Sphere to Tube Force  radius_sphere=link_h/2  radius_tube=flr2_dep/2*(1-0.1)  d_tube=flr2_dep/2*(2*0.1)  l_tube=flr2_wid  active_angle=[-flr2_ang 0]  force_law=Linear  k_contact=flr_k  b_contact=flr_b  pen_full_damp_F=1e-4  pen_exponent=1  custom_param_1=1  custom_param_2=1  friction_law=Stick-Slip Continuous  mu_kinetic=flr_muk  mu_static=flr_mus  v_thr=flr_vth  vis_on=off  vis_opc_en=0  vis_len_tubBx=flr2_dep*flr_dep_pcnt  vis_clr=[0.9 0.2 0.2]  vis_opc=0.7
      settings: SourceProductName=Simscape Multibody Contact Forces Library
  LLeg4 to Edge Force : Contact_Forces_Lib/3D/Sphere to Tube Force  radius_sphere=link_h/2  radius_tube=flr2_dep/2*(1-0.1)  d_tube=flr2_dep/2*(2*0.1)  l_tube=flr2_wid  active_angle=[-flr2_ang 0]  force_law=Linear  k_contact=flr_k  b_contact=flr_b  pen_full_damp_F=1e-4  pen_exponent=1  custom_param_1=1  custom_param_2=1  friction_law=Stick-Slip Continuous  mu_kinetic=flr_muk  mu_static=flr_mus  v_thr=flr_vth  vis_on=off  vis_opc_en=0  vis_len_tubBx=flr2_dep*flr_dep_pcnt  vis_clr=[0.9 0.2 0.2]  vis_opc=0.7
      settings: SourceProductName=Simscape Multibody Contact Forces Library
  RLeg1 to Edge Force : Contact_Forces_Lib/3D/Sphere to Tube Force  radius_sphere=link_h/2  radius_tube=flr2_dep/2*(1-0.1)  d_tube=flr2_dep/2*(2*0.1)  l_tube=flr2_wid  active_angle=[-flr2_ang 0]  force_law=Linear  k_contact=flr_k  b_contact=flr_b  pen_full_damp_F=1e-4  pen_exponent=1  custom_param_1=1  custom_param_2=1  friction_law=Stick-Slip Continuous  mu_kinetic=flr_muk  mu_static=flr_mus  v_thr=flr_vth  vis_on=off  vis_opc_en=0  vis_len_tubBx=flr2_dep*flr_dep_pcnt  vis_clr=[0.9 0.2 0.2]  vis_opc=0.7
      settings: SourceProductName=Simscape Multibody Contact Forces Library
  RLeg23 to Edge Force : Contact_Forces_Lib/3D/Sphere to Tube Force  radius_sphere=link_h/2  radius_tube=flr2_dep/2*(1-0.1)  d_tube=flr2_dep/2*(2*0.1)  l_tube=flr2_wid  active_angle=[-flr2_ang 0]  force_law=Linear  k_contact=flr_k  b_contact=flr_b  pen_full_damp_F=1e-4  pen_exponent=1  custom_param_1=1  custom_param_2=1  friction_law=Stick-Slip Continuous  mu_kinetic=flr_muk  mu_static=flr_mus  v_thr=flr_vth  vis_on=off  vis_opc_en=0  vis_len_tubBx=flr2_dep*flr_dep_pcnt  vis_clr=[0.9 0.2 0.2]  vis_opc=0.7
      settings: SourceProductName=Simscape Multibody Contact Forces Library
  RLeg4 to Edge Force : Contact_Forces_Lib/3D/Sphere to Tube Force  radius_sphere=link_h/2  radius_tube=flr2_dep/2*(1-0.1)  d_tube=flr2_dep/2*(2*0.1)  l_tube=flr2_wid  active_angle=[-flr2_ang 0]  force_law=Linear  k_contact=flr_k  b_contact=flr_b  pen_full_damp_F=1e-4  pen_exponent=1  custom_param_1=1  custom_param_2=1  friction_law=Stick-Slip Continuous  mu_kinetic=flr_muk  mu_static=flr_mus  v_thr=flr_vth  vis_on=off  vis_opc_en=0  vis_len_tubBx=flr2_dep*flr_dep_pcnt  vis_clr=[0.9 0.2 0.2]  vis_opc=0.7
      settings: SourceProductName=Simscape Multibody Contact Forces Library
  Terminator{,1..5} (6 alike) : Terminator
  L4 : PMIOPort  Side=Left
  L23 : PMIOPort  Port=2  Side=Left
  L1 : PMIOPort  Port=3  Side=Left
  R4 : PMIOPort  Port=4  Side=Left
  W : PMIOPort  Port=5  Side=Right
  R23 : PMIOPort  Port=6  Side=Left
  R1 : PMIOPort  Port=7  Side=Left
  wires:
  RLeg1 to Edge Force/1 -> Terminator/1
  LLeg23 to Edge Force/1 -> Terminator4/1
  LLeg4 to Edge Force/1 -> Terminator5/1
  LLeg1 to Edge Force/1 -> Terminator3/1
  RLeg4 to Edge Force/1 -> Terminator2/1
  RLeg23 to Edge Force/1 -> Terminator1/1
  connections:
  LLeg1 to Edge Force/RConn1 -- LLeg23 to Edge Force/RConn1 -- LLeg4 to Edge Force/RConn1 -- W/RConn1 -- Floor/RConn1 -- RLeg23 to Edge Force/RConn1 -- RLeg1 to Edge Force/RConn1 -- RLeg4 to Edge Force/RConn1
  LLeg23 to Edge Force/LConn1 -- L23/RConn1
  RLeg1 to Edge Force/LConn1 -- R1/RConn1
  RLeg23 to Edge Force/LConn1 -- R23/RConn1
  RLeg4 to Edge Force/LConn1 -- R4/RConn1
  LLeg1 to Edge Force/LConn1 -- L1/RConn1
  LLeg4 to Edge Force/LConn1 -- L4/RConn1

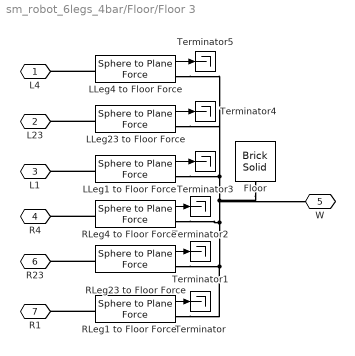
== system sm_robot_6legs_4bar/Floor/Floor 3 ==
  Floor : sm_lib/Body Elements/Brick Solid  BrickDimensions=[flr3_len flr3_wid flr3_dep]  BrickDimensionsUnits=m  ExportEntireGeometry=off  InertiaType=CalculateFromGeometry  BasedOnType=Density  Density=1000  DensityUnits=kg/m^3  Mass=1  MassUnits=kg  CenterOfMass=[0 0 0]  CenterOfMassUnits=m  MomentsOfInertia=[1 1 1]  MomentsOfInertiaUnits=kg*m^2  ProductsOfInertia=[0 0 0]  ProductsOfInertiaUnits=kg*m^2  GraphicType=FromGeometry  MarkerShape=Sphere  MarkerSize=10  GraphicVisPropType=SimpleVisualProperties  GraphicDiffuseColor=flr_clr  GraphicOpacity=1.0  GraphicSpecularColor=[0.5 0.5 0.5 1.0]  GraphicAmbientColor=[0.15 0.15 0.15 1.0]  GraphicEmissiveColor=[0.0 0.0 0.0 1.0]  GraphicShininess=75  DoExposeReferenceFrame=on  SerializedFrames=<Frames/>
  LLeg1 to Floor Force : Contact_Forces_Lib/3D/Sphere to Plane Force  sphere_rad=link_h/2  plane_lenx=flr3_len  plane_leny=flr3_wid  plane_depth=flr3_dep/2  force_law=Linear  k_contact=flr_k  b_contact=flr_b  pen_full_damp_F=1e-4  pen_exponent=1  custom_param_1=1  custom_param_2=1  friction_law=Stick-Slip Continuous  mu_kinetic=flr_muk  mu_static=flr_mus  v_thr=flr_vth  vis_on=off  vis_opc_en=0  vis_len_plaBz=flr3_dep*flr_dep_pcnt  vis_clr=[0.9 0.2 0.2]  vis_opc=0.7
  LLeg23 to Floor Force : Contact_Forces_Lib/3D/Sphere to Plane Force  sphere_rad=link_h/2  plane_lenx=flr3_len  plane_leny=flr3_wid  plane_depth=flr3_dep/2  force_law=Linear  k_contact=flr_k  b_contact=flr_b  pen_full_damp_F=1e-4  pen_exponent=1  custom_param_1=1  custom_param_2=1  friction_law=Stick-Slip Continuous  mu_kinetic=flr_muk  mu_static=flr_mus  v_thr=flr_vth  vis_on=off  vis_opc_en=0  vis_len_plaBz=flr3_dep*flr_dep_pcnt  vis_clr=[0.9 0.2 0.2]  vis_opc=0.7
  LLeg4 to Floor Force : Contact_Forces_Lib/3D/Sphere to Plane Force  sphere_rad=link_h/2  plane_lenx=flr3_len  plane_leny=flr3_wid  plane_depth=flr3_dep/2  force_law=Linear  k_contact=flr_k  b_contact=flr_b  pen_full_damp_F=1e-4  pen_exponent=1  custom_param_1=1  custom_param_2=1  friction_law=Stick-Slip Continuous  mu_kinetic=flr_muk  mu_static=flr_mus  v_thr=flr_vth  vis_on=off  vis_opc_en=0  vis_len_plaBz=flr3_dep*flr_dep_pcnt  vis_clr=[0.9 0.2 0.2]  vis_opc=0.7
  RLeg1 to Floor Force : Contact_Forces_Lib/3D/Sphere to Plane Force  sphere_rad=link_h/2  plane_lenx=flr3_len  plane_leny=flr3_wid  plane_depth=flr3_dep/2  force_law=Linear  k_contact=flr_k  b_contact=flr_b  pen_full_damp_F=1e-4  pen_exponent=1  custom_param_1=1  custom_param_2=1  friction_law=Stick-Slip Continuous  mu_kinetic=flr_muk  mu_static=flr_mus  v_thr=flr_vth  vis_on=off  vis_opc_en=0  vis_len_plaBz=flr3_dep*flr_dep_pcnt  vis_clr=[0.9 0.2 0.2]  vis_opc=0.7
  RLeg23 to Floor Force : Contact_Forces_Lib/3D/Sphere to Plane Force  sphere_rad=link_h/2  plane_lenx=flr3_len  plane_leny=flr3_wid  plane_depth=flr3_dep/2  force_law=Linear  k_contact=flr_k  b_contact=flr_b  pen_full_damp_F=1e-4  pen_exponent=1  custom_param_1=1  custom_param_2=1  friction_law=Stick-Slip Continuous  mu_kinetic=flr_muk  mu_static=flr_mus  v_thr=flr_vth  vis_on=off  vis_opc_en=0  vis_len_plaBz=flr3_dep*flr_dep_pcnt  vis_clr=[0.9 0.2 0.2]  vis_opc=0.7
  RLeg4 to Floor Force : Contact_Forces_Lib/3D/Sphere to Plane Force  sphere_rad=link_h/2  plane_lenx=flr3_len  plane_leny=flr3_wid  plane_depth=flr3_dep/2  force_law=Linear  k_contact=flr_k  b_contact=flr_b  pen_full_damp_F=1e-4  pen_exponent=1  custom_param_1=1  custom_param_2=1  friction_law=Stick-Slip Continuous  mu_kinetic=flr_muk  mu_static=flr_mus  v_thr=flr_vth  vis_on=off  vis_opc_en=0  vis_len_plaBz=flr3_dep*flr_dep_pcnt  vis_clr=[0.9 0.2 0.2]  vis_opc=0.7
  Terminator{,1..5} (6 alike) : Terminator
  L4 : PMIOPort  Side=Left
  L23 : PMIOPort  Port=2  Side=Left
  L1 : PMIOPort  Port=3  Side=Left
  R4 : PMIOPort  Port=4  Side=Left
  W : PMIOPort  Port=5  Side=Right
  R23 : PMIOPort  Port=6  Side=Left
  R1 : PMIOPort  Port=7  Side=Left
  wires:
  RLeg1 to Floor Force/1 -> Terminator/1
  LLeg23 to Floor Force/1 -> Terminator4/1
  LLeg4 to Floor Force/1 -> Terminator5/1
  LLeg1 to Floor Force/1 -> Terminator3/1
  RLeg4 to Floor Force/1 -> Terminator2/1
  RLeg23 to Floor Force/1 -> Terminator1/1
  connections:
  LLeg23 to Floor Force/LConn1 -- L23/RConn1
  RLeg1 to Floor Force/LConn1 -- R1/RConn1
  RLeg23 to Floor Force/LConn1 -- R23/RConn1
  RLeg4 to Floor Force/LConn1 -- R4/RConn1
  LLeg1 to Floor Force/LConn1 -- L1/RConn1
  LLeg4 to Floor Force/LConn1 -- L4/RConn1
  LLeg1 to Floor Force/RConn1 -- W/RConn1 -- Floor/RConn1 -- RLeg23 to Floor Force/RConn1 -- RLeg1 to Floor Force/RConn1 -- RLeg4 to Floor Force/RConn1 -- LLeg23 to Floor Force/RConn1 -- LLeg4 to Floor Force/RConn1

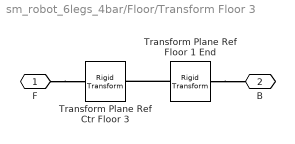
== system sm_robot_6legs_4bar/Floor/Transform Floor 3 ==
  Transform Plane Ref Ctr Floor 3 : sm_lib/Frames and Transforms/Rigid Transform  RotationMethod=None  FollAlignAxisA=+X  BaseAlignAxisA=+Y  FollAlignAxisB=+Y  BaseAlignAxisB=+Z  RotationStandardAxis=+Y  RotationAngle=-10  RotationAngleUnits=deg  RotationArbitraryAxis=[0 0 1]  RotationSequenceAxes=FollowerAxes  RotationSequence=XYX  RotationSequenceAngles=[0 0 0]  RotationSequenceAnglesUnits=deg  RotationMatrix=[1 0 0; 0 1 0; 0 0 1]  Quaternion=[1 0 0 0]  TranslationMethod=Cartesian  TranslationCartesianOffset=[flr3_len/2 0 0]  TranslationCartesianOffsetUnits=m  TranslationStandardAxis=+Z  TranslationStandardOffset=0  TranslationStandardOffsetUnits=m  TranslationROffset=0  TranslationROffsetUnits=m  TranslationThetaOffset=0  TranslationThetaOffsetUnits=deg  TranslationZOffset=0  TranslationZOffsetUnits=m
  Transform Plane Ref Floor 1 End : sm_lib/Frames and Transforms/Rigid Transform  RotationMethod=None  FollAlignAxisA=+X  BaseAlignAxisA=+Y  FollAlignAxisB=+Y  BaseAlignAxisB=+Z  RotationStandardAxis=+Y  RotationAngle=-10  RotationAngleUnits=deg  RotationArbitraryAxis=[0 0 1]  RotationSequenceAxes=FollowerAxes  RotationSequence=XYX  RotationSequenceAngles=[0 0 0]  RotationSequenceAnglesUnits=deg  RotationMatrix=[1 0 0; 0 1 0; 0 0 1]  Quaternion=[1 0 0 0]  TranslationMethod=Cartesian  TranslationCartesianOffset=[cosd(flr2_ang) 0 sind(flr2_ang)]*flr2_len  TranslationCartesianOffsetUnits=m  TranslationStandardAxis=+Z  TranslationStandardOffset=0  TranslationStandardOffsetUnits=m  TranslationROffset=0  TranslationROffsetUnits=m  TranslationThetaOffset=0  TranslationThetaOffsetUnits=deg  TranslationZOffset=0  TranslationZOffsetUnits=m
  F : PMIOPort  Side=Right
  B : PMIOPort  Port=2  Side=Left
  connections:
  Transform Plane Ref Floor 1 End/RConn1 -- Transform Plane Ref Ctr Floor 3/LConn1
  Transform Plane Ref Floor 1 End/LConn1 -- B/RConn1
  F/RConn1 -- Transform Plane Ref Ctr Floor 3/RConn1
